simulink model "LQR_pendulum_model"  (R2024b)
settings: Solver=ode3  StartTime=0.0  StopTime=t(end)  RelTol=1e-3
undefined symbols (not defined in the file): fi_dc0, g, J_pend, J_rotor, K, kr, kt, omega_dc0, omega_pend0, R, U, uc_dc, uc_pend, uv_dc, uv_pend
settings Model: Creator=Student  LastModifiedBy=Paweł Wiktor
settings SolverCC: AlgebraicLoopSolver=TrustRegion
settings DataIOCC: ReturnWorkspaceOutputs=off
settings DebuggingCC: UnconnectedInputMsg=warning  UnconnectedOutputMsg=warning  UnconnectedLineMsg=warning  ArithmeticOperatorsInVariantConditions=warning
settings ModelReferenceCC: EnableRefExpFcnMdlSchedulingChecks=on
settings SFSimCC: CustomCodeUndefinedFunction=UseInterfaceOnly
settings RTWCC: GPUComputeCapability=3.5

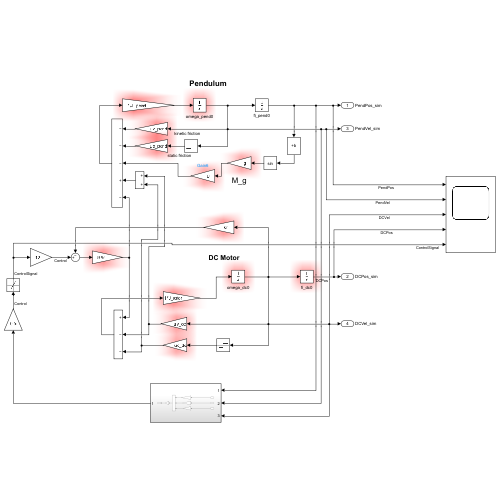
[thumbnail: Simulink's stored preview of the top-level diagram]
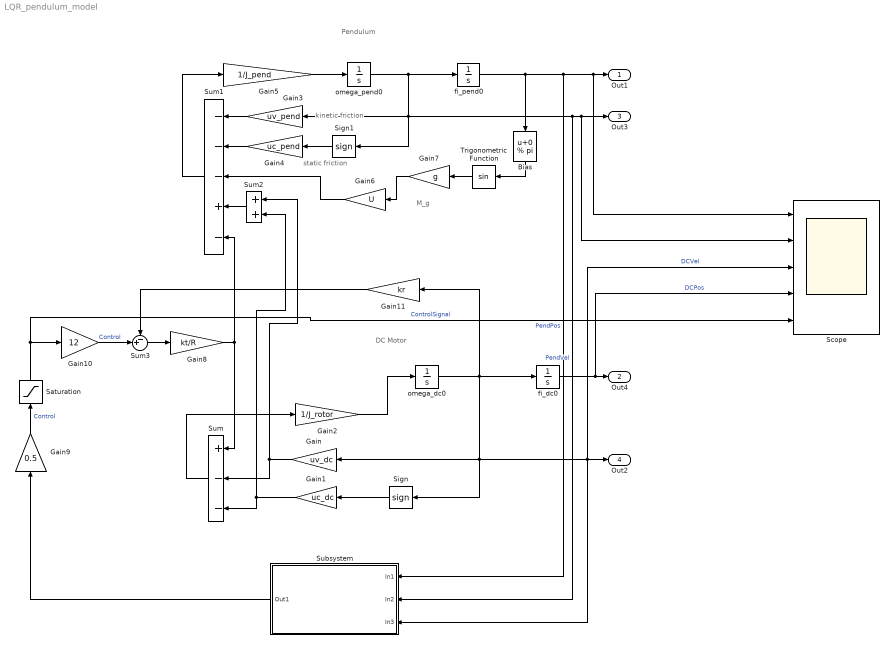
== system LQR_pendulum_model ==
  note: DC Motor
  note: Pendulum
  note: kinetic friction
  note: static friction
  note: M_g
  Bias : Bias  Bias=0 % pi  SaturateOnIntegerOverflow=off
  Gain : Gain  Gain=uv_dc
  Gain1 : Gain  Gain=uc_dc
  Gain10 : Gain  Gain=12
  Gain11 : Gain  Gain=kr
  Gain2 : Gain  Gain=1/J_rotor
  Gain3 : Gain  Gain=uv_pend
  Gain4 : Gain  Gain=uc_pend
  Gain5 : Gain  Gain=1/J_pend
  Gain6 : Gain  Gain=U
  Gain7 : Gain  Gain=g
  Gain8 : Gain  Gain=kt/R
  Gain9 : Gain  Gain=0.5
  Saturation : Saturate  UpperLimit=1  LowerLimit=-1
  Scope : Scope  NumInputPorts=5
  Sign : Signum  ZeroCross=off
  Sign1 : Signum  ZeroCross=off
  Subsystem : Subsystem
  Sum : Sum  Inputs=+--
  Sum1 : Sum  Inputs=---+-
  Sum2 : Sum
  Sum3 : Sum  Inputs=-+|
  Trigonometric Function : Trigonometry
  fi_dc0 : Integrator  InitialCondition=fi_dc0
  fi_pend0 : Integrator  InitialCondition=0.5
  omega_dc0 : Integrator  InitialCondition=omega_dc0
  omega_pend0 : Integrator  InitialCondition=omega_pend0
  Out1 : Outport  SignalName=PendPos_sim  VectorParamsAs1DForOutWhenUnconnected=off
  Out4 : Outport  Port=2  SignalName=DCPos_sim  VectorParamsAs1DForOutWhenUnconnected=off
  Out3 : Outport  Port=3  SignalName=PendVel_sim  VectorParamsAs1DForOutWhenUnconnected=off
  Out2 : Outport  Port=4  SignalName=DCVel_sim  VectorParamsAs1DForOutWhenUnconnected=off
  wires:
  omega_dc0/1 -> Gain11/1, fi_dc0/1, Scope/3, Subsystem/3(In3), Out2/1, Sign/1, Gain/1  "DCVel"
  Gain2/1 -> omega_dc0/1
  Sum/1 -> Gain2/1
  Sign/1 -> Gain1/1
  Gain6/1 -> Sum1/3
  Gain7/1 -> Gain6/1
  Sum1/1 -> Gain5/1
  omega_pend0/1 -> Sign1/1, Subsystem/2(In2), Scope/2, Out3/1, Gain3/1, fi_pend0/1  "PendVel"
  Gain3/1 -> Sum1/1
  Trigonometric Function/1 -> Gain7/1
  fi_pend0/1 -> Subsystem/1(In1), Scope/1, Out1/1, Bias/1  "PendPos"
  Sign1/1 -> Gain4/1
  Gain5/1 -> omega_pend0/1
  Gain4/1 -> Sum1/2
  fi_dc0/1 -> Scope/4, Out4/1  "DCPos"
  Gain8/1 -> Sum1/5, Sum/1
  Gain1/1 -> Sum/3, Sum2/2
  Gain/1 -> Sum/2, Sum2/1
  Sum2/1 -> Sum1/4
  Gain9/1 -> Saturation/1  "Control"
  Gain10/1 -> Sum3/2  "Control"
  Saturation/1 -> Scope/5, Gain10/1  "ControlSignal"
  Sum3/1 -> Gain8/1
  Gain11/1 -> Sum3/1
  Bias/1 -> Trigonometric Function/1
  Subsystem/1(Out1) -> Gain9/1

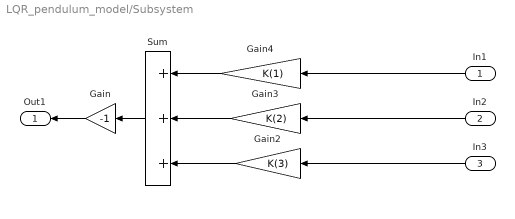
== system LQR_pendulum_model/Subsystem ==
  In1 : Inport
  In2 : Inport  Port=2
  In3 : Inport  Port=3
  Gain : Gain  Gain=-1
  Gain2 : Gain  Gain=K(3)
  Gain3 : Gain  Gain=K(2)
  Gain4 : Gain  Gain=K(1)
  Sum : Sum  Inputs=+++
  Out1 : Outport  VectorParamsAs1DForOutWhenUnconnected=off
  wires:
  In1/1 -> Gain4/1
  In2/1 -> Gain3/1
  In3/1 -> Gain2/1
  Gain2/1 -> Sum/3
  Gain3/1 -> Sum/2
  Gain4/1 -> Sum/1
  Sum/1 -> Gain/1
  Gain/1 -> Out1/1
